simulink library "Input_Tyfocor_LS"  (Simulink 8.2)
settings: Solver=ode45  StartTime=0.0  StopTime=10.0  RelTol=1e-3
settings Model: Creator=lena.frank  LastModifiedBy=drhf

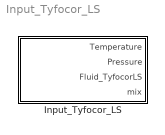
== system Input_Tyfocor_LS ==
  Input_Tyfocor_LS : Subsystem  mask(Input_Tyfocor_LS){T=20, p=1e5}
      mask prompts: T "temperature (scalar or vector) [°C]"; p "pressure [Pa]"
      mask help:
      | Input block for the material "Tyfocor_LS". The relevant inputs for the calculation of the block can be specified as parameter in the mask.
      | Tyfocor is a registered trademark of Tyforop Chemie, Hamburg (Germany).
      mask Help: web(fullfile(path_carnot('help'),'input_material.html'),'-helpbrowser')

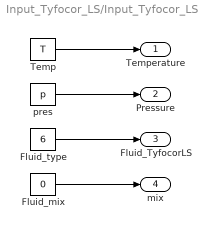
== system Input_Tyfocor_LS/Input_Tyfocor_LS ==
  Fluid_mix : Constant  Value=0
  Fluid_type : Constant  Value=6
  Temp : Constant  Value=T
  pres : Constant  Value=p
  Temperature : Outport
  Pressure : Outport  Port=2
  Fluid_TyfocorLS : Outport  Port=3
  mix : Outport  Port=4
  wires:
  Fluid_mix/1 -> mix/1
  Fluid_type/1 -> Fluid_TyfocorLS/1
  Temp/1 -> Temperature/1
  pres/1 -> Pressure/1
